simulink model "quad_nonlinearmpc"  (R2017a)
settings: Solver=ode113  StartTime=0.0  StopTime=50  MaxStep=0.2  MinStep=0.01  RelTol=1e-3
undefined symbols (not defined in the file or in its folder): magnitude
settings Model: SimulationMode=accelerator  Creator=sherief nabeeh  LastModifiedBy=sherief nabeeh
settings SolverCC: SolverResetMethod=Robust
settings OptimizationCC: EfficientMapNaN2IntZero=off
settings HardwareCC: TargetBitPerPointer=64  TargetBitPerSizeT=64  TargetBitPerPtrDiffT=64  TargetLongLongMode=on  TargetIntDivRoundTo=Zero  TargetEndianess=LittleEndian  TargetWordSize=64  TargetHWDeviceType=MATLAB Host  ProdEqTarget=off
settings CodeAppCC: MaxIdLength=128
settings GRTTargetCC: TargetLangStandard=C89/C90 (ANSI)  CombineOutputUpdateFcns=off  GRTInterface=on  UseToolchainInfoCompliant=off

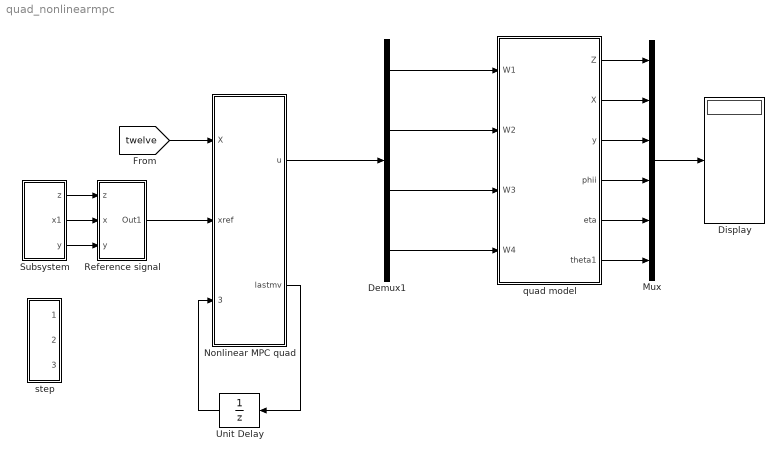
== system quad_nonlinearmpc ==
  Demux1 : Demux
  Display : Display
  Mux : Mux  Inputs=6
  Nonlinear MPC quad : MATLAB Function  TreatAsAtomicUnit=on
  Reference signal : Subsystem
  Subsystem : Subsystem
  Unit Delay : UnitDelay  SampleTime=-1
  quad model : Subsystem
  step : Subsystem
  wires:
  Demux1/1 -> quad model/1(W1)
  Demux1/2 -> quad model/2(W2)
  Demux1/3 -> quad model/3(W3)
  Demux1/4 -> quad model/4(W4)
  Nonlinear MPC quad/1(u) -> Demux1/1
  Nonlinear MPC quad/2(lastmv) -> Unit Delay/1
  Unit Delay/1 -> Nonlinear MPC quad/3(lastmv_in)
  quad model/1(Z) -> Mux/1
  quad model/2(X) -> Mux/2
  quad model/3(y) -> Mux/3
  quad model/4(phii) -> Mux/4
  quad model/5(eta) -> Mux/5
  quad model/6(theta1) -> Mux/6
  [twelve] -> Nonlinear MPC quad/1(X)
  Reference signal/1(Out1) -> Nonlinear MPC quad/2(xref)
  Mux/1 -> Display/1
  Subsystem/1(z) -> Reference signal/1(z)
  Subsystem/2(x1) -> Reference signal/2(x)
  Subsystem/3(y) -> Reference signal/3(y)

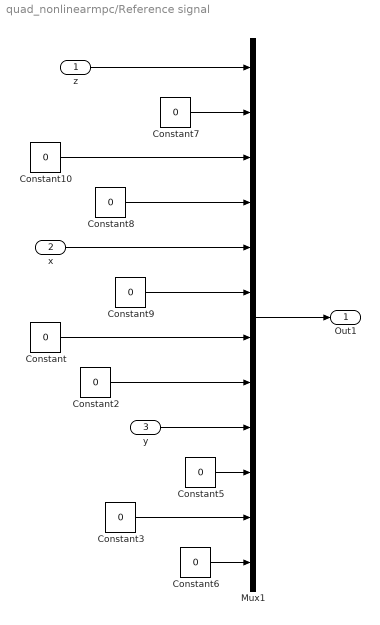
== system quad_nonlinearmpc/Reference signal ==
  z : Inport
  x : Inport  Port=2
  y : Inport  Port=3
  Constant{,2..3,5..10} (9 alike) : Constant  Value=0
  Mux1 : Mux  Inputs=12
  Out1 : Outport
  wires:
  z/1 -> Mux1/1
  Constant7/1 -> Mux1/2
  Constant8/1 -> Mux1/4
  Constant9/1 -> Mux1/6
  Constant10/1 -> Mux1/3
  x/1 -> Mux1/5
  Mux1/1 -> Out1/1
  Constant/1 -> Mux1/7
  Constant2/1 -> Mux1/8
  y/1 -> Mux1/9
  Constant6/1 -> Mux1/12
  Constant3/1 -> Mux1/11
  Constant5/1 -> Mux1/10

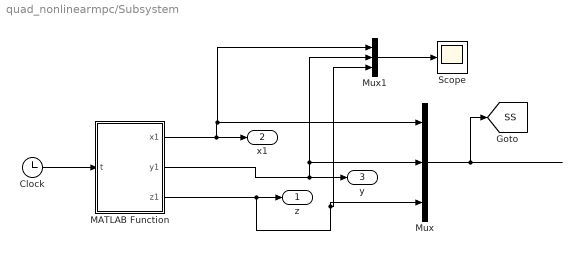
== system quad_nonlinearmpc/Subsystem ==
  Clock : Clock
  MATLAB Function : MATLAB Function  TreatAsAtomicUnit=on
  Mux : Mux  Inputs=3
  Mux1 : Mux  Inputs=3
  Scope : Scope
  z : Outport
  x1 : Outport  Port=2
  y : Outport  Port=3
  tag scope: SS=global
  wires:
  MATLAB Function/2(y1) -> Mux1/2, Mux/2, y/1
  MATLAB Function/3(z1) -> Mux1/3, Mux/3, z/1
  Clock/1 -> MATLAB Function/1(t)
  MATLAB Function/1(x1) -> x1/1, Mux1/1, Mux/1
  Mux/1 -> [SS]
  Mux1/1 -> Scope/1

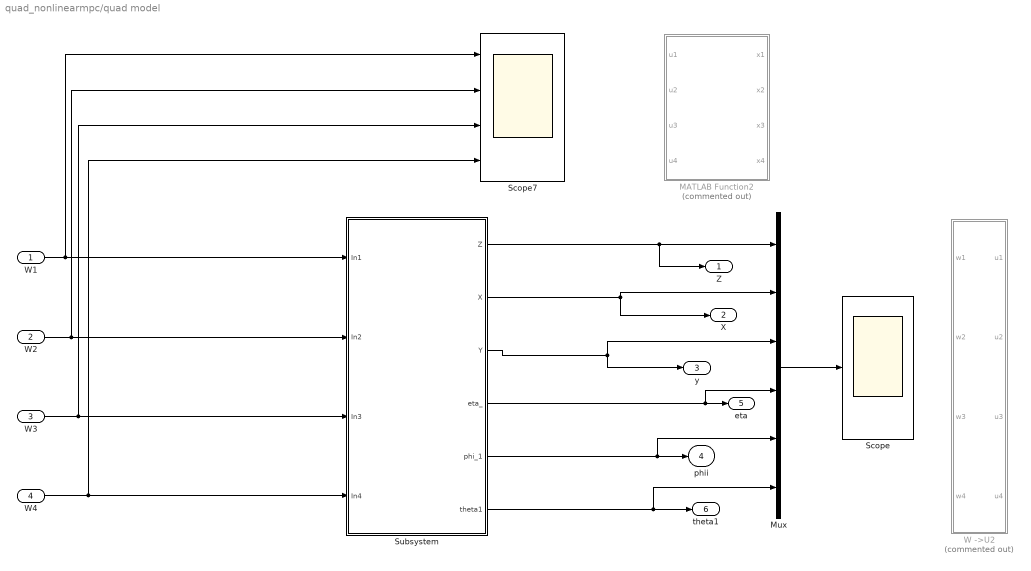
== system quad_nonlinearmpc/quad model ==
  W1 : Inport
  W2 : Inport  Port=2
  W3 : Inport  Port=3
  W4 : Inport  Port=4
  MATLAB Function2 : MATLAB Function  Commented=on  TreatAsAtomicUnit=on
  Mux : Mux  Inputs=6
  Scope : Scope
  Scope7 : Scope  NumInputPorts=4
  Subsystem : Subsystem
  W ->U2 : Subsystem  Commented=on
  Z : Outport
  X : Outport  Port=2
  y : Outport  Port=3
  phii : Outport  Port=4
  eta : Outport  Port=5
  theta1 : Outport  Port=6
  wires:
  Subsystem/1(Z) -> Z/1, Mux/1
  Subsystem/3(Y) -> Mux/3, y/1
  Subsystem/5(phi_1) -> Mux/5, phii/1
  Subsystem/6(theta1) -> Mux/6, theta1/1
  Subsystem/4(eta_) -> Mux/4, eta/1
  Subsystem/2(X) -> Mux/2, X/1
  Mux/1 -> Scope/1
  W1/1 -> Subsystem/1(In1), Scope7/1
  W2/1 -> Subsystem/2(In2), Scope7/2
  W3/1 -> Subsystem/3(In3), Scope7/3
  W4/1 -> Subsystem/4(In4), Scope7/4

== system quad_nonlinearmpc/step ==
  Step1 : Step  Time=0  After=3  SampleTime=0
  Step2 : Step  Time=0  SampleTime=0
  Step3 : Step  Time=0  After=3  SampleTime=0
  Out1 : Outport
  Out2 : Outport  Port=2
  Out3 : Outport  Port=3
  wires:
  Step2/1 -> Out1/1
  Step1/1 -> Out2/1
  Step3/1 -> Out3/1

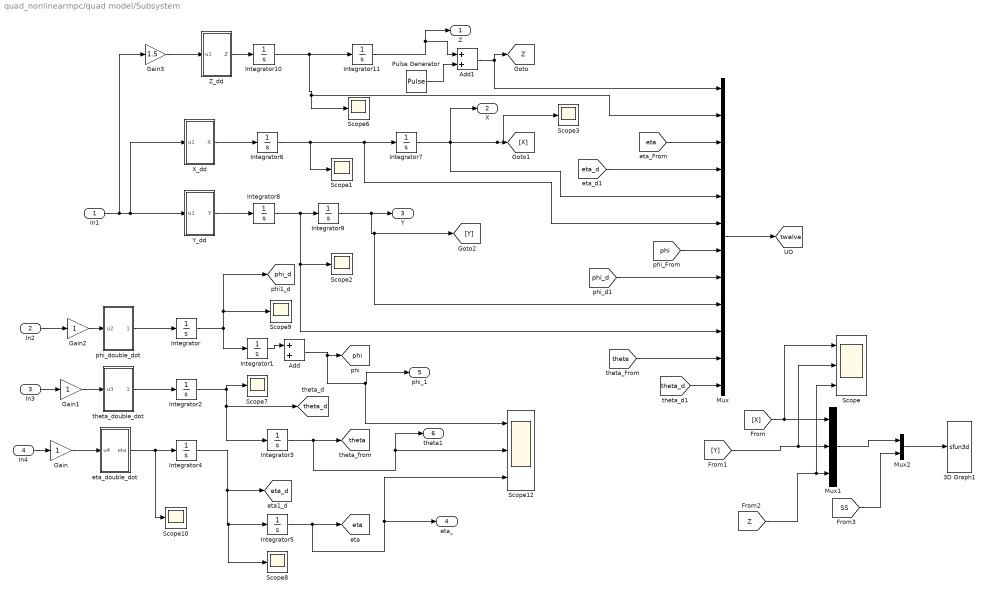
== system quad_nonlinearmpc/quad model/Subsystem ==
  In1 : Inport
  In2 : Inport  Port=2
  In3 : Inport  Port=3
  In4 : Inport  Port=4
  3D Graph1 : S-Function  LoadFcn=if exist('sfun3d','file'), sfun3d([],[],[],'LoadBlock'); end  FunctionName=sfun3d  Parameters=ax,T,np,cp,gd,ls,mk,mx,hd,tb  SFunctionDeploymentMode=off  EnableBusSupport=off  mask(3D Graph){np=2, ax=[-7 7 -7 7 0 50], mx=100000, T=0.05, cp=[370 -234 -207], gd=on, hd=off, tb=on, ls=-, mk=none}
      mask prompts: np "Number of moving points (lines)"; ax "Range: [xmin xmax  ymin ymax zmin zmax]"; mx "Max number of points in each line"; T "Sampling Time"; cp "Camera position (use [0 0 1] for 2D XY view)"; gd "Grid (on|off)"; hd "HeadMarkers (on|off)"; tb "Toolbar (on|off)"; ls "LineStyle"; mk "LineMarker"
      mask help:
      | This block plots the position of several points in the XYZ space. The input contains the coordinates of all the points (x1,y1,z1,x2,y2,z2,...).
      | The number of moving points (lines), the XYZ ranges, sampling time, camera position, and grid (among other things) can be set as mask parameters.
      settings: CopyFcn=if exist('sfun3d','file'), sfun3d([],[],[],'CopyBlock'); end  DeleteFcn=if exist('sfun3d','file'), sfun3d([],[],[],'DeleteBlock'); end  NameChangeFcn=if exist('sfun3d','file'), sfun3d([],[],[],'NameChange'); end
      mask Help:
      | This block plots the position of several points in the XYZ space. The input contains the coordinates of all the points (x1,y1,z1,x2,y2,z2,...).
      | The number of moving points (lines), the XYZ ranges, sampling time, camera position, and grid (among other things) can be set as mask parameters.
      mask TypeOptions ls: - | -- | : | -. | none
      mask TypeOptions mk: none | . | + | o | * | x | square | diamond | v | ^ | > | < | pentagram | hexagram
      mask Display: plot([.05 .95 .95 .05 .05],[.45 .45 .95 .95 .45], 0.5+cos(0:0.1:2*pi)*0.3,0.7+sin(0:0.1:2*pi)*0.2)
  Add : Sum
  Add1 : Sum
  Gain : Gain
  Gain1 : Gain
  Gain2 : Gain
  Gain3 : Gain  Gain=1.5
  Integrator{,1..11} (12 alike) : Integrator
  Mux : Mux  Inputs=12
  Mux1 : Mux  Inputs=3
  Mux2 : Mux  Inputs=2
  Pulse Generator : DiscretePulseGenerator  PulseType=Time based  Amplitude=-4  Period=1  PulseWidth=99  PhaseDelay=8
  Scope : Scope  NumInputPorts=3
  Scope{1..3,6..10} (8 alike) : Scope
  Scope12 : Scope  NumInputPorts=3
  "X_dd " : Subsystem
  Y_dd : Subsystem
  Z_dd : Subsystem
  eta_double_dot : Subsystem
  phi_double_dot : Subsystem
  theta_double_dot : Subsystem
  Z : Outport
  X : Outport  Port=2
  Y : Outport  Port=3
  eta_ : Outport  Port=4
  phi_1 : Outport  Port=5
  theta1 : Outport  Port=6
  tag scope: Z=global, eta=global, eta_d=global, phi=global, phi_d=global, theta=global, theta_d=global, twelve=global
  wires:
  Integrator11/1 -> Add1/1, Z/1
  eta_double_dot/1(eta) -> Scope10/1, Integrator4/1
  In4/1 -> Gain/1
  Integrator6/1 -> Scope1/1, Mux/6, Integrator7/1
  Integrator7/1 -> Scope3/1, [X], Mux/5, X/1
  Integrator2/1 -> Integrator3/1, [theta_d], Scope7/1
  Integrator/1 -> Scope9/1, [phi_d], Integrator1/1
  phi_double_dot/1(phi_) -> Integrator/1
  In2/1 -> Gain2/1
  Integrator4/1 -> Scope8/1, Integrator5/1, [eta_d]
  "X_dd "/1(X) -> Integrator6/1
  Y_dd/1(Y) -> Integrator8/1
  In3/1 -> Gain1/1
  Integrator9/1 -> Y/1, [Y], Mux/9
  In1/1 -> Y_dd/1(u1), "X_dd "/1(u1), Gain3/1
  Z_dd/1(Z) -> Integrator10/1
  Integrator3/1 -> Scope12/2, theta1/1, [theta]
  Integrator5/1 -> Scope12/3, eta_/1, [eta]
  theta_double_dot/1(theta) -> Integrator2/1
  Mux/1 -> [twelve]
  Integrator10/1 -> Mux/2, Scope6/1, Integrator11/1
  [eta] -> Mux/3
  [eta_d] -> Mux/4
  [phi] -> Mux/7
  [phi_d] -> Mux/8
  Integrator8/1 -> Scope2/1, Mux/10, Integrator9/1
  [theta] -> Mux/11
  [theta_d] -> Mux/12
  Gain/1 -> eta_double_dot/1(u4)
  Gain1/1 -> theta_double_dot/1(u3)
  Gain2/1 -> phi_double_dot/1(u2)
  [Y] -> Scope/2, Mux1/2
  [Z] -> Scope/3, Mux1/3
  [X] -> Scope/1, Mux1/1
  Gain3/1 -> Z_dd/1(u1)
  Mux2/1 -> 3D Graph1/1
  Mux1/1 -> Mux2/1
  [SS] -> Mux2/2
  Add/1 -> Scope12/1, phi_1/1, [phi]
  Integrator1/1 -> Add/1
  Add1/1 -> [Z], Mux/1
  Pulse Generator/1 -> Add1/2

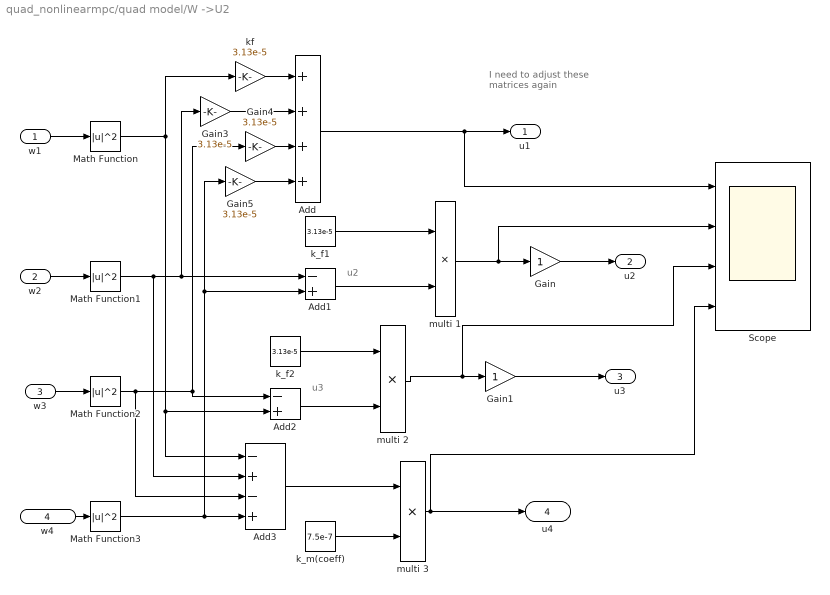
== system quad_nonlinearmpc/quad model/W ->U2 ==
  note: I need to adjust these matrices again
  note: u2
  note: u3
  w1 : Inport
  w2 : Inport  Port=2
  w3 : Inport  Port=3
  w4 : Inport  Port=4
  Add : Sum  Inputs=++++
  Add1 : Sum  Inputs=-+
  Add2 : Sum  Inputs=-+
  Add3 : Sum  Inputs=-+-+
  Gain : Gain
  Gain1 : Gain
  Gain3 : Gain  Gain=3.13e-5
  Gain4 : Gain  Gain=3.13e-5
  Gain5 : Gain  Gain=3.13e-5
  Math Function{,1..3} (4 alike) : Math  Operator=magnitude^2  SaturateOnIntegerOverflow=on
  Scope : Scope  NumInputPorts=4
  k_f1 : Constant  Value=3.13e-5
  k_f2 : Constant  Value=3.13e-5
  k_m(coeff) : Constant  Value=7.5e-7
  kf : Gain  Gain=3.13e-5
  multi 1 : Product  Inputs=**
  multi 2 : Product  Inputs=**
  multi 3 : Product  Inputs=**
  u1 : Outport
  "u2 " : Outport  Port=2
  u3 : Outport  Port=3
  u4 : Outport  Port=4
  wires:
  Add/1 -> u1/1, Scope/1
  multi 3/1 -> Scope/4, u4/1
  k_f2/1 -> multi 2/1
  Add2/1 -> multi 2/2
  multi 2/1 -> Scope/3, Gain1/1
  Add3/1 -> multi 3/1
  Math Function2/1 -> Add3/3, Add2/1, Gain4/1
  Math Function1/1 -> Add3/2, Add1/1, Gain3/1
  Math Function3/1 -> Add1/2, Gain5/1, Add3/4
  multi 1/1 -> Scope/2, Gain/1
  k_m(coeff)/1 -> multi 3/2
  Math Function/1 -> Add3/1, Add2/2, kf/1
  k_f1/1 -> multi 1/1
  Add1/1 -> multi 1/2
  kf/1 -> Add/1
  Gain3/1 -> Add/2
  Gain4/1 -> Add/3
  Gain5/1 -> Add/4
  w4/1 -> Math Function3/1
  w3/1 -> Math Function2/1
  w2/1 -> Math Function1/1
  w1/1 -> Math Function/1
  Gain/1 -> "u2 "/1
  Gain1/1 -> u3/1

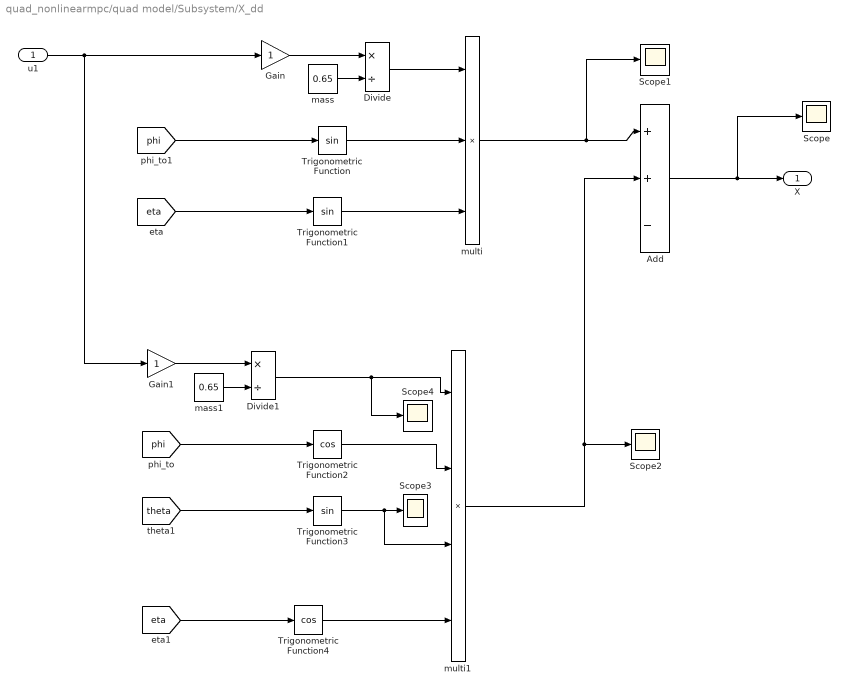
== system quad_nonlinearmpc/quad model/Subsystem/X_dd  ==
  u1 : Inport
  Add : Sum  Inputs=++-
  Divide : Product  Inputs=*/
  Divide1 : Product  Inputs=*/
  Gain : Gain
  Gain1 : Gain
  Scope{,1..4} (5 alike) : Scope
  Trigonometric Function : Trigonometry
  Trigonometric Function1 : Trigonometry
  Trigonometric Function2 : Trigonometry  Operator=cos
  Trigonometric Function3 : Trigonometry
  Trigonometric Function4 : Trigonometry  Operator=cos
  mass : Constant  Value=0.65
  mass1 : Constant  Value=0.65
  multi : Product  Inputs=***
  multi1 : Product  Inputs=****
  X : Outport
  wires:
  multi/1 -> Scope1/1, Add/1
  Add/1 -> Scope/1, X/1
  mass/1 -> Divide/2
  Gain/1 -> Divide/1
  multi1/1 -> Scope2/1, Add/2
  Trigonometric Function2/1 -> multi1/2
  Trigonometric Function3/1 -> multi1/3, Scope3/1
  Divide/1 -> multi/1
  Trigonometric Function/1 -> multi/2
  Trigonometric Function1/1 -> multi/3
  [phi] -> Trigonometric Function/1
  [eta] -> Trigonometric Function1/1
  [phi] -> Trigonometric Function2/1
  [theta] -> Trigonometric Function3/1
  mass1/1 -> Divide1/2
  Gain1/1 -> Divide1/1
  u1/1 -> Gain1/1, Gain/1
  Divide1/1 -> Scope4/1, multi1/1
  Trigonometric Function4/1 -> multi1/4
  [eta] -> Trigonometric Function4/1

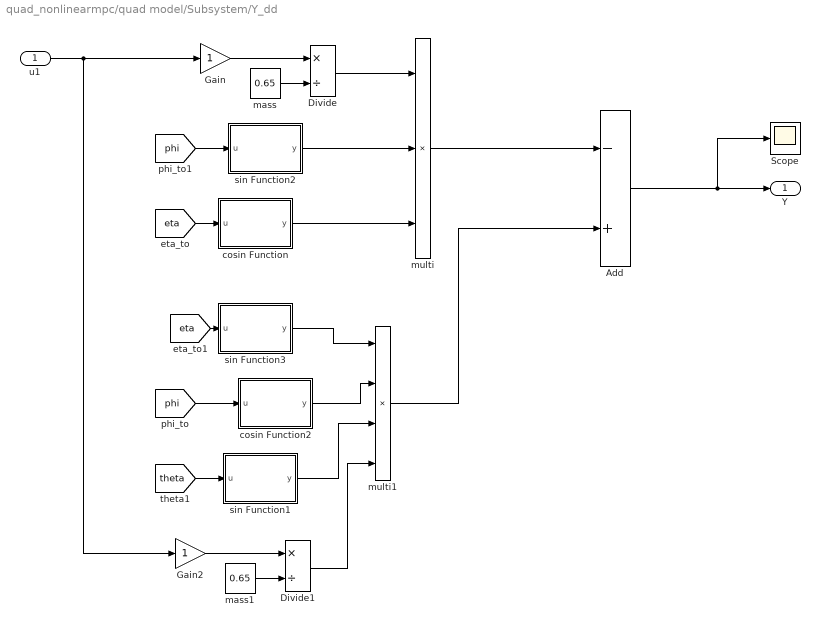
== system quad_nonlinearmpc/quad model/Subsystem/Y_dd ==
  u1 : Inport
  Add : Sum  Inputs=-+
  Divide : Product  Inputs=*/
  Divide1 : Product  Inputs=*/
  Gain : Gain
  Gain2 : Gain
  Scope : Scope
  cosin Function : MATLAB Function  TreatAsAtomicUnit=on
  cosin Function2 : MATLAB Function  TreatAsAtomicUnit=on
  mass : Constant  Value=0.65
  mass1 : Constant  Value=0.65
  multi : Product  Inputs=***
  multi1 : Product  Inputs=****
  sin Function1 : MATLAB Function  TreatAsAtomicUnit=on
  sin Function2 : MATLAB Function  TreatAsAtomicUnit=on
  sin Function3 : MATLAB Function  TreatAsAtomicUnit=on
  Y : Outport
  wires:
  multi/1 -> Add/1
  Add/1 -> Scope/1, Y/1
  mass/1 -> Divide/2
  Gain/1 -> Divide/1
  [eta] -> cosin Function/1(u)
  multi1/1 -> Add/2
  [theta] -> sin Function1/1(u)
  [phi] -> cosin Function2/1(u)
  cosin Function2/1(y) -> multi1/2
  sin Function1/1(y) -> multi1/3
  Divide/1 -> multi/1
  cosin Function/1(y) -> multi/3
  sin Function2/1(y) -> multi/2
  [phi] -> sin Function2/1(u)
  mass1/1 -> Divide1/2
  Gain2/1 -> Divide1/1
  Divide1/1 -> multi1/4
  u1/1 -> Gain2/1, Gain/1
  sin Function3/1(y) -> multi1/1
  [eta] -> sin Function3/1(u)

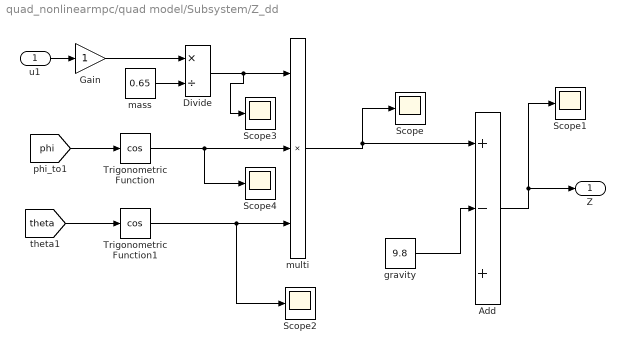
== system quad_nonlinearmpc/quad model/Subsystem/Z_dd ==
  u1 : Inport
  Add : Sum  Inputs=+-+
  Divide : Product  Inputs=*/
  Gain : Gain
  Scope{,1..4} (5 alike) : Scope
  Trigonometric Function : Trigonometry  Operator=cos
  Trigonometric Function1 : Trigonometry  Operator=cos
  gravity : Constant  Value=9.8
  mass : Constant  Value=0.65
  multi : Product  Inputs=***
  Z : Outport
  wires:
  u1/1 -> Gain/1
  multi/1 -> Scope/1, Add/1
  Add/1 -> Scope1/1, Z/1
  mass/1 -> Divide/2
  Gain/1 -> Divide/1
  [theta] -> Trigonometric Function1/1
  gravity/1 -> Add/2
  Trigonometric Function1/1 -> Scope2/1, multi/3
  [phi] -> Trigonometric Function/1
  Divide/1 -> Scope3/1, multi/1
  Trigonometric Function/1 -> Scope4/1, multi/2

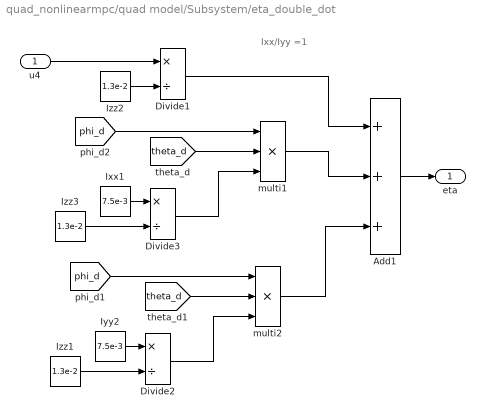
== system quad_nonlinearmpc/quad model/Subsystem/eta_double_dot ==
  note: Ixx/Iyy =1
  u4 : Inport
  Add1 : Sum  Inputs=+++
  Divide1 : Product  Inputs=*/
  Divide2 : Product  Inputs=*/
  Divide3 : Product  Inputs=*/
  Ixx1 : Constant  Value=7.5e-3
  Iyy2 : Constant  Value=7.5e-3
  Izz1 : Constant  Value=1.3e-2
  Izz2 : Constant  Value=1.3e-2
  Izz3 : Constant  Value=1.3e-2
  multi1 : Product  Inputs=***
  multi2 : Product  Inputs=***
  eta : Outport
  wires:
  Izz2/1 -> Divide1/2
  Divide2/1 -> multi2/3
  [phi_d] -> multi2/1
  [theta_d] -> multi2/2
  Divide3/1 -> multi1/3
  Izz3/1 -> Divide3/2
  Ixx1/1 -> Divide3/1
  [phi_d] -> multi1/1
  [theta_d] -> multi1/2
  Izz1/1 -> Divide2/2
  Iyy2/1 -> Divide2/1
  multi2/1 -> Add1/3
  multi1/1 -> Add1/2
  Divide1/1 -> Add1/1
  Add1/1 -> eta/1
  u4/1 -> Divide1/1

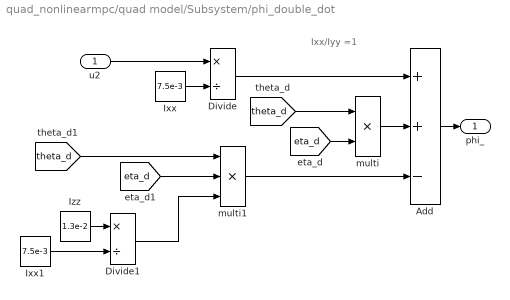
== system quad_nonlinearmpc/quad model/Subsystem/phi_double_dot ==
  note: Ixx/Iyy =1
  u2 : Inport
  Add : Sum  Inputs=++-
  Divide : Product  Inputs=*/
  Divide1 : Product  Inputs=*/
  Ixx : Constant  Value=7.5e-3
  Ixx1 : Constant  Value=7.5e-3
  Izz : Constant  Value=1.3e-2
  multi : Product  Inputs=**
  multi1 : Product  Inputs=***
  phi_ : Outport
  wires:
  Divide/1 -> Add/1
  u2/1 -> Divide/1
  multi/1 -> Add/2
  Add/1 -> phi_/1
  [theta_d] -> multi/1
  Ixx/1 -> Divide/2
  [eta_d] -> multi/2
  multi1/1 -> Add/3
  Divide1/1 -> multi1/3
  Ixx1/1 -> Divide1/2
  Izz/1 -> Divide1/1
  [theta_d] -> multi1/1
  [eta_d] -> multi1/2

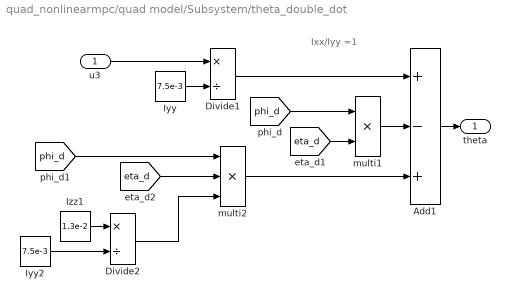
== system quad_nonlinearmpc/quad model/Subsystem/theta_double_dot ==
  note: Ixx/Iyy =1
  u3 : Inport
  Add1 : Sum  Inputs=+-+
  Divide1 : Product  Inputs=*/
  Divide2 : Product  Inputs=*/
  Iyy : Constant  Value=7.5e-3
  Iyy2 : Constant  Value=7.5e-3
  Izz1 : Constant  Value=1.3e-2
  multi1 : Product  Inputs=**
  multi2 : Product  Inputs=***
  theta : Outport
  wires:
  Divide1/1 -> Add1/1
  u3/1 -> Divide1/1
  multi1/1 -> Add1/2
  Add1/1 -> theta/1
  [phi_d] -> multi1/1
  Iyy/1 -> Divide1/2
  [eta_d] -> multi1/2
  multi2/1 -> Add1/3
  Divide2/1 -> multi2/3
  Iyy2/1 -> Divide2/2
  Izz1/1 -> Divide2/1
  [phi_d] -> multi2/1
  [eta_d] -> multi2/2

== matlab function quad_nonlinearmpc/Nonlinear MPC quad ==
  data: X input; xref input; u output; lastmv_in input; lastmv output
function [u,lastmv] = fcn(X,xref,lastmv_in)

% Implementation of Nonlinear MPC (for simulation only)
coder.extrinsic('quad_optim','fprintf','tic','toc')
% control interval
Ts = 0.01;
% prediction horizon
N = 10;
% online references (velocity references are always zero)
% xref = [0;0;0;0;5;0;0;0;5;0;0;0];
% nonlinear mpc computation
lastmv = zeros(4,N); % must initialize uopt because of extrinsic function 
[lastmv,n] = quad_optim(X,xref,Ts,N,lastmv_in);    
% optimal move
u = lastmv(:,1);

fprintf('%d',n);
% fprintf('%d',J);

== matlab function quad_nonlinearmpc/quad model/MATLAB Function2 ==
  data: x1 output; x2 output; x3 output; x4 output; u1 input; u2 input; u3 input; u4 input
function [x1, x2, x3, x4] =fcn(u1, u2, u3, u4)

coder.extrinsic('myfcn');
w1=0;
w2=0;
w3=0;
w4=0;

[w1,w2,w3,w4]= myfcn(u1,u2,u3,u4);
x1 = w1;
x2 =w2; 
x3=w3;
x4=w4;

== matlab function quad_nonlinearmpc/quad model/Subsystem/Y_dd/sin Function3 ==
  data: u input; y output
function y = fcn(u)
%#codegen

y = sin(u);

== matlab function quad_nonlinearmpc/Subsystem/MATLAB Function ==
  data: t input; x1 output; y1 output; z1 output
function [x1,y1,z1] = fcn(t)

x1=3*cos(0.4*t)
 y1=3*sin(0.4*t)
 z1=0.9*t

== matlab function quad_nonlinearmpc/quad model/Subsystem/Y_dd/cosin Function ==
  data: u input; y output
function y = fcn(u)
%#codegen

y = cos(u);

== matlab function quad_nonlinearmpc/quad model/Subsystem/Y_dd/sin Function2 ==
  data: u input; y output
function y = fcn(u)
%#codegen

y = sin(u);

== matlab function quad_nonlinearmpc/quad model/Subsystem/Y_dd/sin Function1 ==
  data: u input; y output
function y = fcn(u)
%#codegen

y = sin(u);

== matlab function quad_nonlinearmpc/quad model/Subsystem/Y_dd/cosin Function2 ==
  data: u input; y output
function y = fcn(u)
%#codegen

y = cos(u);
